simulink model "SystemPIDClosedLoop_motor_closed_zrate_js"  (Simulink 7.7)
settings: Solver=ode4  StartTime=0.0  StopTime=60  FixedStep=0.001  RelTol=1e-3
libraries: simulink x5, aerolibanimutils x1, aerolibfltsims x1
settings Model: Creator=Rakhi  LastModifiedBy=Rakhi
settings SolverCC: PositivePriorityOrder=on

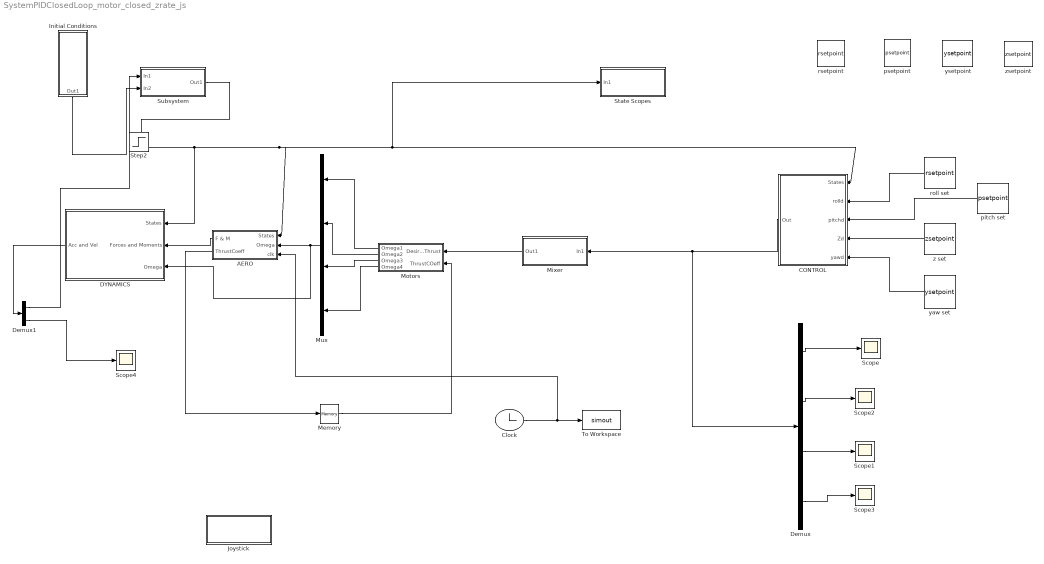
== system SystemPIDClosedLoop_motor_closed_zrate_js ==
  AERO : Subsystem
  CONTROL : Subsystem
      settings: AttributesFormatString=%<Priority>
  Clock : Clock
  DYNAMICS : Subsystem
  Demux : Demux
  Demux1 : Demux  Outputs=[12 1]
  Initial Conditions : Subsystem
  Joystick : Subsystem
  Memory : Memory  X0=3.1751e-5  InheritSampleTime=on
  Mixer : Subsystem
  Motors : Subsystem
  Mux : Mux
  Scope{,1..4} (5 alike) : Scope
      Scope settings: YMin=-900  YMax=-50
      Scope1 settings: YMin=-30  YMax=30
      Scope2 settings: SaveName=ScopeData2
      Scope3 settings: SaveName=ScopeData3
      Scope4 settings: SaveName=ScopeData4
  State Scopes : Subsystem
  Subsystem : Subsystem
  To Workspace : ToWorkspace  VariableName=simout  SampleTime=-1  SaveFormat=Structure
      settings: MaxDataPoints=1
  pitch set : DataStoreRead  DataStoreName=psetpoint  SampleTime=0.001  DataStoreElements=psetpoint
  psetpoint : DataStoreMemory  DataStoreName=psetpoint
  roll set : DataStoreRead  DataStoreName=rsetpoint  SampleTime=0.001  DataStoreElements=rsetpoint
  rsetpoint : DataStoreMemory  DataStoreName=rsetpoint
  yaw set : DataStoreRead  DataStoreName=ysetpoint  SampleTime=0.001  DataStoreElements=ysetpoint
  ysetpoint : DataStoreMemory  DataStoreName=ysetpoint
  z set : DataStoreRead  DataStoreName=zsetpoint  SampleTime=0.001  DataStoreElements=zsetpoint
  zsetpoint : DataStoreMemory  DataStoreName=zsetpoint  InitialValue=-45
  Step2 : Step  IOType=siggen  SampleTime=0
  wires:
  AERO/1(F & M) -> DYNAMICS/2(Forces and Moments)
  Initial Conditions/1(Out1) -> Subsystem/2(In2)
  Subsystem/1(Out1) -> DYNAMICS/1(States), AERO/1(States), CONTROL/1(States), State Scopes/1(In1)
  Demux/1 -> Scope/1
  Demux/2 -> Scope2/1
  Demux/4 -> Scope3/1
  CONTROL/1(Out) -> Mixer/1(In1), Demux/1
  Demux1/1 -> Subsystem/1(In1)
  DYNAMICS/1(Acc and Vel) -> Demux1/1
  Demux1/2 -> Scope4/1
  Clock/1 -> To Workspace/1, AERO/3(clk)
  Mux/1 -> AERO/2(Omega), DYNAMICS/3(Omega)
  Demux/3 -> Scope1/1
  AERO/2(ThrustCoeff) -> Memory/1
  Mixer/1(Out1) -> Motors/1(DesiredThrust)
  Memory/1 -> Motors/2(ThrustCOeff)
  Motors/1(Omega1) -> Mux/1
  Motors/2(Omega2) -> Mux/2
  Motors/3(Omega3) -> Mux/3
  Motors/4(Omega4) -> Mux/4
  roll set/1 -> CONTROL/2(rolld)
  pitch set/1 -> CONTROL/3(pitchd)
  z set/1 -> CONTROL/4(Zd)
  yaw set/1 -> CONTROL/5(yawd)

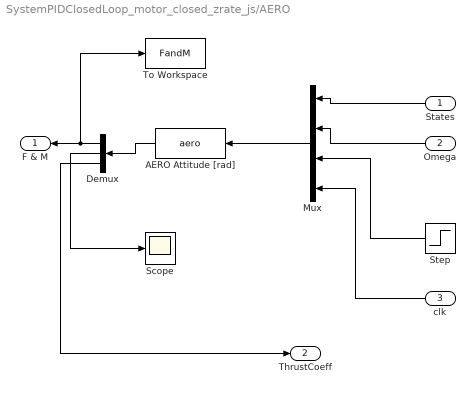
== system SystemPIDClosedLoop_motor_closed_zrate_js/AERO ==
  States : Inport
  Omega : Inport  Port=2
  clk : Inport  Port=3
  AERO Attitude [rad] : MATLABFcn  MATLABFcn=aero  OutputDimensions=26
  Demux : Demux  Outputs=[24 1 1]
  Mux : Mux
  Scope : Scope
      settings: SaveName=ScopeData5
  Step : Step  Time=0  Before=4  After=4  SampleTime=0
  To Workspace : ToWorkspace  VariableName=FandM  SampleTime=-1  SaveFormat=Structure
      settings: MaxDataPoints=1
  F & M : Outport
  ThrustCoeff : Outport  Port=2
  wires:
  Step/1 -> Mux/3
  Omega/1 -> Mux/2
  States/1 -> Mux/1
  Mux/1 -> AERO Attitude [rad]/1
  clk/1 -> Mux/4
  AERO Attitude [rad]/1 -> Demux/1
  Demux/1 -> F & M/1, To Workspace/1
  Demux/2 -> Scope/1
  Demux/3 -> ThrustCoeff/1

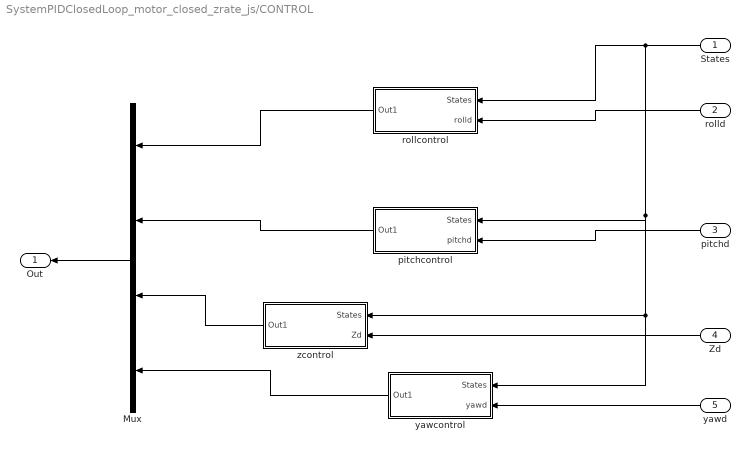
== system SystemPIDClosedLoop_motor_closed_zrate_js/CONTROL ==
  States : Inport
  rolld : Inport  Port=2
  pitchd : Inport  Port=3
  Zd : Inport  Port=4
  yawd : Inport  Port=5
  Mux : Mux
  pitchcontrol : Subsystem
  rollcontrol : Subsystem
  yawcontrol : Subsystem
  zcontrol : Subsystem
  Out : Outport
  wires:
  States/1 -> rollcontrol/1(States), pitchcontrol/1(States), yawcontrol/1(States), zcontrol/1(States)
  rolld/1 -> rollcontrol/2(rolld)
  pitchd/1 -> pitchcontrol/2(pitchd)
  yawd/1 -> yawcontrol/2(yawd)
  Zd/1 -> zcontrol/2(Zd)
  rollcontrol/1(Out1) -> Mux/1
  pitchcontrol/1(Out1) -> Mux/2
  zcontrol/1(Out1) -> Mux/3
  yawcontrol/1(Out1) -> Mux/4
  Mux/1 -> Out/1

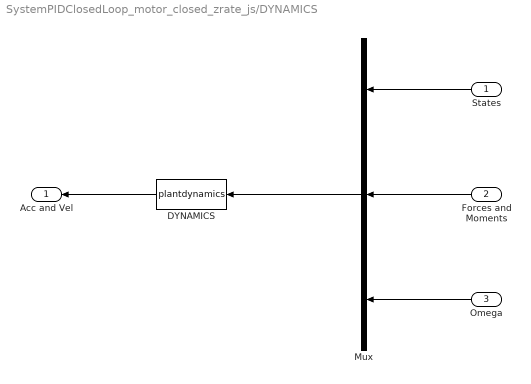
== system SystemPIDClosedLoop_motor_closed_zrate_js/DYNAMICS ==
  States : Inport
  Forces and Moments : Inport  Port=2
  Omega : Inport  Port=3
  DYNAMICS : MATLABFcn  MATLABFcn=plantdynamics  OutputDimensions=13
  Mux : Mux  Inputs=3
  Acc and Vel : Outport
  wires:
  States/1 -> Mux/1
  Forces and Moments/1 -> Mux/2
  Omega/1 -> Mux/3
  Mux/1 -> DYNAMICS/1
  DYNAMICS/1 -> Acc and Vel/1

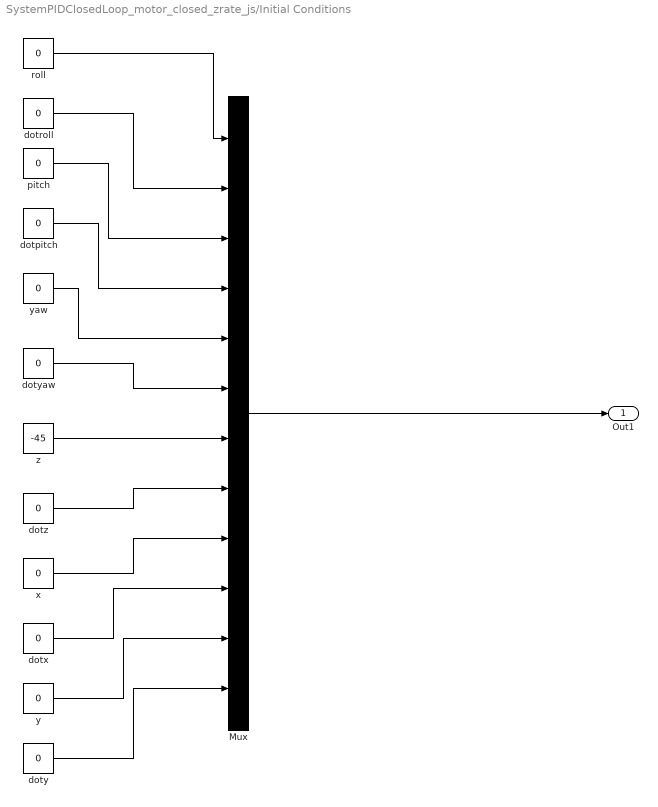
== system SystemPIDClosedLoop_motor_closed_zrate_js/Initial Conditions ==
  Mux : Mux  Inputs=12
  dotpitch : Constant  Value=0
  dotroll : Constant  Value=0
  dotx : Constant  Value=0
  doty : Constant  Value=0
  dotyaw : Constant  Value=0
  dotz : Constant  Value=0
  pitch : Constant  Value=0
  roll : Constant  Value=0
  x : Constant  Value=0
  y : Constant  Value=0
  yaw : Constant  Value=0
  z : Constant  Value=-45
  Out1 : Outport
  wires:
  doty/1 -> Mux/12
  y/1 -> Mux/11
  dotx/1 -> Mux/10
  x/1 -> Mux/9
  dotz/1 -> Mux/8
  z/1 -> Mux/7
  dotyaw/1 -> Mux/6
  yaw/1 -> Mux/5
  dotpitch/1 -> Mux/4
  pitch/1 -> Mux/3
  dotroll/1 -> Mux/2
  roll/1 -> Mux/1
  Mux/1 -> Out1/1

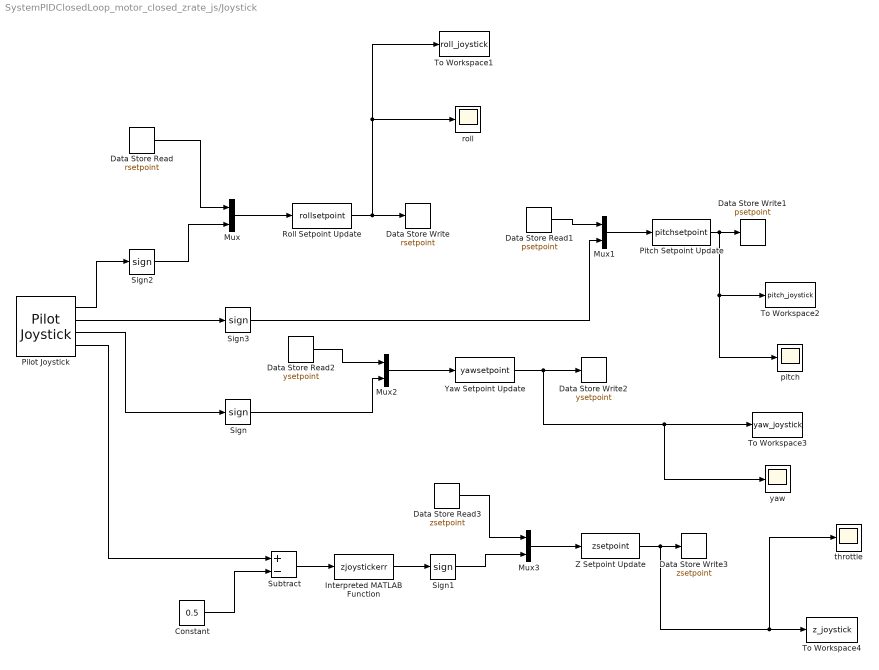
== system SystemPIDClosedLoop_motor_closed_zrate_js/Joystick ==
  Constant : Constant  Value=0.5
  Data Store Read : DataStoreRead  DataStoreName=rsetpoint  SampleTime=0.001  DataStoreElements=rsetpoint
  Data Store Read1 : DataStoreRead  DataStoreName=psetpoint  SampleTime=0.001  DataStoreElements=psetpoint
  Data Store Read2 : DataStoreRead  DataStoreName=ysetpoint  SampleTime=0.001  DataStoreElements=ysetpoint
  Data Store Read3 : DataStoreRead  DataStoreName=zsetpoint  SampleTime=.001  DataStoreElements=zsetpoint
  Data Store Write : DataStoreWrite  DataStoreName=rsetpoint  SampleTime=0.001  DataStoreElements=rsetpoint
  Data Store Write1 : DataStoreWrite  DataStoreName=psetpoint  SampleTime=0.001  DataStoreElements=psetpoint
  Data Store Write2 : DataStoreWrite  DataStoreName=ysetpoint  SampleTime=0.001  DataStoreElements=ysetpoint
  Data Store Write3 : DataStoreWrite  DataStoreName=zsetpoint  SampleTime=.001  DataStoreElements=zsetpoint
  Interpreted MATLAB Function : MATLABFcn  MATLABFcn=zjoystickerr
  Mux{,1..3} (4 alike) : Mux  Inputs=2
  Pilot Joystick : aerolibanimutils/Pilot Joystick  JoystickID=Joystick1  OutputConfiguration=FourAxis  SampleTime=0.001
  Pitch Setpoint Update : MATLABFcn  MATLABFcn=pitchsetpoint
  Roll Setpoint Update : MATLABFcn  MATLABFcn=rollsetpoint
  Sign{,1..3} (4 alike) : Signum
  Subtract : Sum  Inputs=+-
  To Workspace1 : ToWorkspace  VariableName=roll_joystick  SampleTime=-1  SaveFormat=Array
      settings: MaxDataPoints=1
  To Workspace2 : ToWorkspace  VariableName=pitch_joystick  SampleTime=-1  SaveFormat=Array
      settings: MaxDataPoints=1
  To Workspace3 : ToWorkspace  VariableName=yaw_joystick  SampleTime=-1  SaveFormat=Array
      settings: MaxDataPoints=1
  To Workspace4 : ToWorkspace  VariableName=z_joystick  SampleTime=-1  SaveFormat=Array
      settings: MaxDataPoints=1
  Yaw Setpoint Update : MATLABFcn  MATLABFcn=yawsetpoint
  Z Setpoint Update : MATLABFcn  MATLABFcn=zsetpoint
  pitch : Scope
      settings: YMin=-1  YMax=1  SaveName=ScopeData19
  roll : Scope
      settings: YMin=-1.5  YMax=1.5  SaveName=ScopeData21
  throttle : Scope
      settings: YMin=-49.5  YMax=-42.5  SaveName=ScopeData22
  yaw : Scope
      settings: YMin=-1.5  YMax=1.5  SaveName=ScopeData23
  wires:
  Pilot Joystick/3 -> Sign/1
  Constant/1 -> Subtract/2
  Pilot Joystick/4 -> Subtract/1
  Subtract/1 -> Interpreted MATLAB Function/1
  Interpreted MATLAB Function/1 -> Sign1/1
  Pilot Joystick/1 -> Sign2/1
  Pilot Joystick/2 -> Sign3/1
  Mux/1 -> Roll Setpoint Update/1
  Data Store Read/1 -> Mux/1
  Sign2/1 -> Mux/2
  Roll Setpoint Update/1 -> Data Store Write/1, To Workspace1/1, roll/1
  Data Store Read1/1 -> Mux1/1
  Sign3/1 -> Mux1/2
  Mux1/1 -> Pitch Setpoint Update/1
  Pitch Setpoint Update/1 -> Data Store Write1/1, To Workspace2/1, pitch/1
  Data Store Read2/1 -> Mux2/1
  Sign/1 -> Mux2/2
  Mux2/1 -> Yaw Setpoint Update/1
  Yaw Setpoint Update/1 -> Data Store Write2/1, To Workspace3/1, yaw/1
  Sign1/1 -> Mux3/2
  Data Store Read3/1 -> Mux3/1
  Mux3/1 -> Z Setpoint Update/1
  Z Setpoint Update/1 -> Data Store Write3/1, To Workspace4/1, throttle/1

== system SystemPIDClosedLoop_motor_closed_zrate_js/Mixer ==
  In1 : Inport
  Interpreted MATLAB Function : MATLABFcn  MATLABFcn=mix  OutputDimensions=4
  Out1 : Outport
  wires:
  In1/1 -> Interpreted MATLAB Function/1
  Interpreted MATLAB Function/1 -> Out1/1

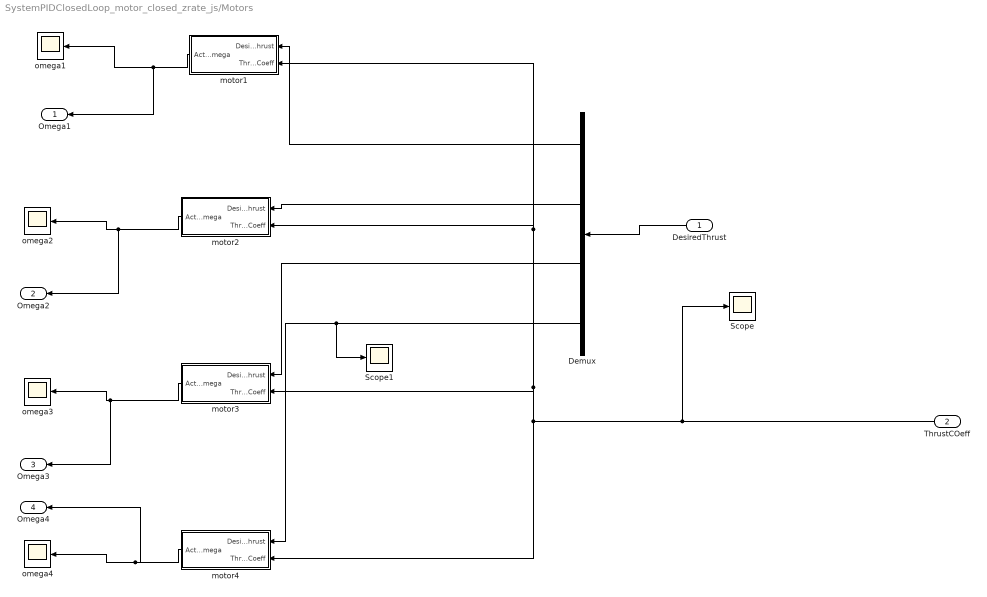
== system SystemPIDClosedLoop_motor_closed_zrate_js/Motors ==
  DesiredThrust : Inport
  ThrustCOeff : Inport  Port=2
  Demux : Demux
  Scope : Scope
      settings: SaveName=ScopeData7
  Scope1 : Scope
      settings: SaveName=ScopeData26
  motor1 : Subsystem
  motor2 : Subsystem
  motor3 : Subsystem
  motor4 : Subsystem
  omega{1..4} (4 alike) : Scope
      omega1 settings: YMin=-1  SaveName=ScopeData9
      omega2 settings: YMax=1  SaveName=ScopeData11
      omega3 settings: YMax=1  SaveName=ScopeData18
      omega4 settings: YMax=1  SaveName=ScopeData20
  Omega1 : Outport
  Omega2 : Outport  Port=2
  Omega3 : Outport  Port=3
  Omega4 : Outport  Port=4
  wires:
  DesiredThrust/1 -> Demux/1
  motor1/1(Actual Omega) -> Omega1/1, omega1/1
  motor2/1(Actual Omega) -> omega2/1, Omega2/1
  motor3/1(Actual Omega) -> omega3/1, Omega3/1
  motor4/1(Actual Omega) -> omega4/1, Omega4/1
  Demux/1 -> motor1/1(DesiredThrust)
  ThrustCOeff/1 -> motor1/2(ThrustCoeff), motor2/2(ThrustCoeff), motor3/2(ThrustCoeff), motor4/2(ThrustCoeff), Scope/1
  Demux/2 -> motor2/1(DesiredThrust)
  Demux/3 -> motor3/1(DesiredThrust)
  Demux/4 -> motor4/1(DesiredThrust), Scope1/1

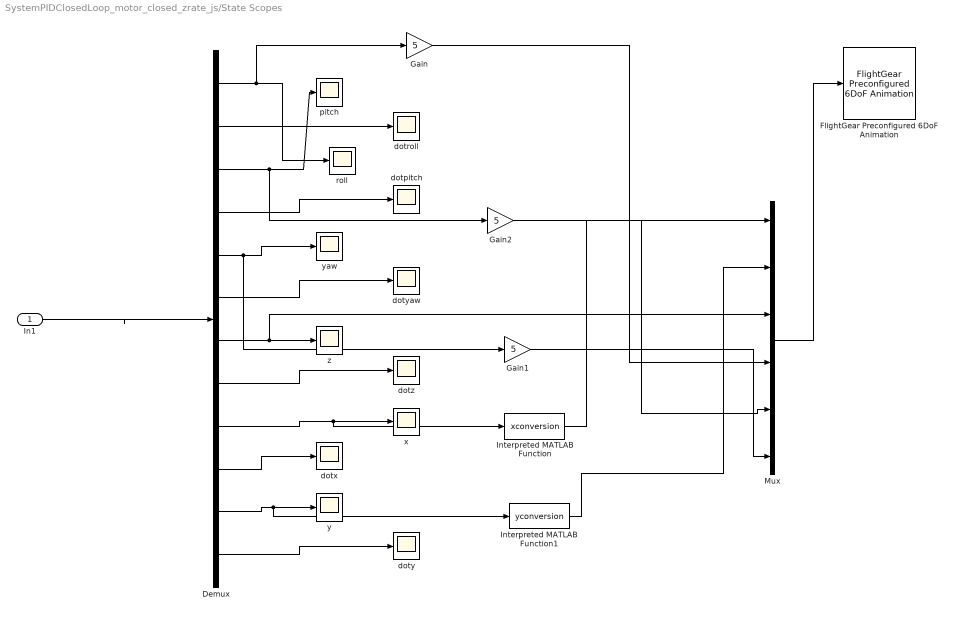
== system SystemPIDClosedLoop_motor_closed_zrate_js/State Scopes ==
  In1 : Inport
  Demux : Demux  Outputs=12
  FlightGear Preconfigured 6DoF Animation : aerolibfltsims/FlightGear Preconfigured 6DoF Animation  SystemSampleTime=-1  xFlightGearVersion=v0.9.8  DestinationIpAddress=127.0.0.1  DestinationPort=5502  SampleTime=-1
  Gain : Gain  Gain=5
  Gain1 : Gain  Gain=5
  Gain2 : Gain  Gain=5
  Interpreted MATLAB Function : MATLABFcn  MATLABFcn=xconversion
  Interpreted MATLAB Function1 : MATLABFcn  MATLABFcn=yconversion
  Mux : Mux  Inputs=6
  dotpitch : Scope
      settings: SaveName=ScopeData8
  dotroll : Scope
      settings: SaveName=ScopeData6
  dotx : Scope
      settings: SaveName=ScopeData14
  doty : Scope
      settings: SaveName=ScopeData16
  dotyaw : Scope
      settings: SaveName=ScopeData10
  dotz : Scope
      settings: SaveName=ScopeData12
  pitch : Scope
      settings: YMin=-0.5  YMax=0.5  SaveName=sc_pitch  DataFormat=Array
  roll : Scope
      settings: YMin=-0.0325  YMax=0  SaveName=sc_roll  DataFormat=Array
  x : Scope
      settings: SaveName=ScopeData13
  y : Scope
      settings: TimeRange=0.7999999999999972  YMin=-470.8125  YMax=-454.8125  SaveName=ScopeData15
  yaw : Scope
      settings: YMin=-0.5  YMax=0.1  SaveName=sc_yaw  DataFormat=Array
  z : Scope
      settings: YMin=-45  YMax=-44.2  SaveName=sc_z  DataFormat=Array
  wires:
  In1/1 -> Demux/1
  Demux/1 -> roll/1, Gain/1
  Demux/2 -> dotroll/1
  Demux/3 -> pitch/1, Gain2/1
  Demux/4 -> dotpitch/1
  Demux/5 -> yaw/1, Gain1/1
  Demux/6 -> dotyaw/1
  Demux/7 -> Mux/3, z/1
  Demux/8 -> dotz/1
  Demux/9 -> x/1, Interpreted MATLAB Function/1
  Demux/10 -> dotx/1
  Demux/11 -> y/1, Interpreted MATLAB Function1/1
  Demux/12 -> doty/1
  Interpreted MATLAB Function1/1 -> Mux/2
  Interpreted MATLAB Function/1 -> Mux/1
  Mux/1 -> FlightGear Preconfigured 6DoF Animation/1
  Gain/1 -> Mux/4
  Gain2/1 -> Mux/5
  Gain1/1 -> Mux/6

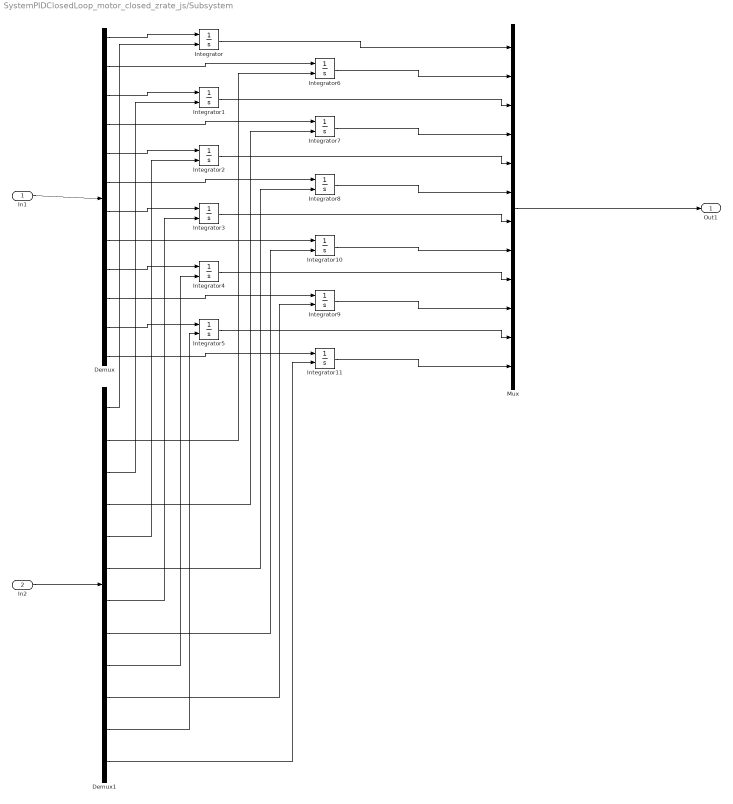
== system SystemPIDClosedLoop_motor_closed_zrate_js/Subsystem ==
  In1 : Inport
  In2 : Inport  Port=2
  Demux : Demux  Outputs=12
  Demux1 : Demux  Outputs=12
  Integrator{,1..11} (12 alike) : Integrator  InitialConditionSource=external
  Mux : Mux  Inputs=12
  Out1 : Outport
  wires:
  Demux/1 -> Integrator/1
  Demux/2 -> Integrator6/1
  Demux/3 -> Integrator1/1
  Demux/4 -> Integrator7/1
  Demux/5 -> Integrator2/1
  Demux/6 -> Integrator8/1
  Demux/7 -> Integrator3/1
  Demux/8 -> Integrator10/1
  Demux/9 -> Integrator4/1
  Demux/10 -> Integrator9/1
  Demux/11 -> Integrator5/1
  Demux/12 -> Integrator11/1
  In1/1 -> Demux/1
  Demux1/1 -> Integrator/2
  Demux1/2 -> Integrator6/2
  Demux1/3 -> Integrator1/2
  Demux1/4 -> Integrator7/2
  Demux1/5 -> Integrator2/2
  Demux1/6 -> Integrator8/2
  Demux1/7 -> Integrator3/2
  Demux1/8 -> Integrator10/2
  Demux1/9 -> Integrator4/2
  Demux1/10 -> Integrator9/2
  Demux1/11 -> Integrator5/2
  Demux1/12 -> Integrator11/2
  In2/1 -> Demux1/1
  Integrator/1 -> Mux/1
  Integrator6/1 -> Mux/2
  Integrator1/1 -> Mux/3
  Integrator7/1 -> Mux/4
  Integrator2/1 -> Mux/5
  Integrator8/1 -> Mux/6
  Integrator3/1 -> Mux/7
  Integrator10/1 -> Mux/8
  Integrator4/1 -> Mux/9
  Integrator9/1 -> Mux/10
  Integrator5/1 -> Mux/11
  Integrator11/1 -> Mux/12
  Mux/1 -> Out1/1

== system SystemPIDClosedLoop_motor_closed_zrate_js/CONTROL/pitchcontrol ==
  States : Inport
  pitchd : Inport  Port=2
  Interpreted MATLAB Function : MATLABFcn  MATLABFcn=pitcherr  OutputDimensions=1
  Mux : Mux  Inputs=2
  PID Controller : simulink/Continuous/PID Controller  SystemSampleTime=-1  Controller=PID  TimeDomain=Continuous-time  SampleTime=1  IntegratorMethod=Forward Euler  FilterMethod=Forward Euler  Form=Parallel  P=0.005  I=0  D=0.025  N=25  InitialConditionSource=internal  InitialConditionForIntegrator=0  InitialConditionForFilter=0  ExternalReset=none  LimitOutput=off  UpperSaturationLimit=inf  LowerSaturationLimit=-inf  LinearizeAsGain=off  AntiWindupMode=none  Kb=1  TrackingMode=off  Kt=1  PParamMin=[]  PParamMax=[]  IParamMin=[]  IParamMax=[]  DParamMin=[]  DParamMax=[]  NParamMin=[]  NParamMax=[]  KbParamMin=[]  KbParamMax=[]  KtParamMin=[]  KtParamMax=[]  POutMin=[]  POutMax=[]  IOutMin=[]  IOutMax=[]  DOutMin=[]  DOutMax=[]  NOutMin=[]  NOutMax=[]  KbOutMin=[]  KbOutMax=[]  KtOutMin=[]  KtOutMax=[]  IntegratorOutMin=[]  IntegratorOutMax=[]  FilterOutMin=[]  FilterOutMax=[]  SumOutMin=[]  SumOutMax=[]  SumI1OutMin=[]  SumI1OutMax=[]  SumI2OutMin=[]  SumI2OutMax=[]  SumI3OutMin=[]  SumI3OutMax=[]  SumDOutMin=[]  SumDOutMax=[]  SaturationOutMin=[]  SaturationOutMax=[]  IntegratorContinuousStateAttributes=''  IntegratorStateMustResolveToSignalObject=off  IntegratorRTWStateStorageClass=Auto  FilterContinuousStateAttributes=''  FilterStateMustResolveToSignalObject=off  FilterRTWStateStorageClass=Auto
  Out1 : Outport
  wires:
  States/1 -> Mux/1
  pitchd/1 -> Mux/2
  Mux/1 -> Interpreted MATLAB Function/1
  Interpreted MATLAB Function/1 -> PID Controller/1
  PID Controller/1 -> Out1/1

== system SystemPIDClosedLoop_motor_closed_zrate_js/CONTROL/rollcontrol ==
  States : Inport
  rolld : Inport  Port=2
  Interpreted MATLAB Function : MATLABFcn  MATLABFcn=rollerr  OutputDimensions=1
  Mux : Mux  Inputs=2
  PID Controller : simulink/Continuous/PID Controller  SystemSampleTime=-1  Controller=PID  TimeDomain=Continuous-time  SampleTime=1  IntegratorMethod=Forward Euler  FilterMethod=Forward Euler  Form=Parallel  P=.005  I=0  D=.025  N=25  InitialConditionSource=internal  InitialConditionForIntegrator=0  InitialConditionForFilter=0  ExternalReset=none  LimitOutput=off  UpperSaturationLimit=inf  LowerSaturationLimit=-inf  LinearizeAsGain=off  AntiWindupMode=none  Kb=1  TrackingMode=off  Kt=1  PParamMin=[]  PParamMax=[]  IParamMin=[]  IParamMax=[]  DParamMin=[]  DParamMax=[]  NParamMin=[]  NParamMax=[]  KbParamMin=[]  KbParamMax=[]  KtParamMin=[]  KtParamMax=[]  POutMin=[]  POutMax=[]  IOutMin=[]  IOutMax=[]  DOutMin=[]  DOutMax=[]  NOutMin=[]  NOutMax=[]  KbOutMin=[]  KbOutMax=[]  KtOutMin=[]  KtOutMax=[]  IntegratorOutMin=[]  IntegratorOutMax=[]  FilterOutMin=[]  FilterOutMax=[]  SumOutMin=[]  SumOutMax=[]  SumI1OutMin=[]  SumI1OutMax=[]  SumI2OutMin=[]  SumI2OutMax=[]  SumI3OutMin=[]  SumI3OutMax=[]  SumDOutMin=[]  SumDOutMax=[]  SaturationOutMin=[]  SaturationOutMax=[]  IntegratorContinuousStateAttributes=''  IntegratorStateMustResolveToSignalObject=off  IntegratorRTWStateStorageClass=Auto  FilterContinuousStateAttributes=''  FilterStateMustResolveToSignalObject=off  FilterRTWStateStorageClass=Auto
  Out1 : Outport
  wires:
  States/1 -> Mux/1
  rolld/1 -> Mux/2
  Mux/1 -> Interpreted MATLAB Function/1
  Interpreted MATLAB Function/1 -> PID Controller/1
  PID Controller/1 -> Out1/1

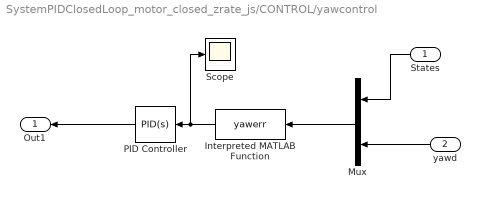
== system SystemPIDClosedLoop_motor_closed_zrate_js/CONTROL/yawcontrol ==
  States : Inport
  yawd : Inport  Port=2
  Interpreted MATLAB Function : MATLABFcn  MATLABFcn=yawerr  OutputDimensions=1
  Mux : Mux  Inputs=2
  PID Controller : simulink/Continuous/PID Controller  SystemSampleTime=-1  Controller=PID  TimeDomain=Continuous-time  SampleTime=1  IntegratorMethod=Forward Euler  FilterMethod=Forward Euler  Form=Parallel  P=0.05  I=0  D=0.25  N=25  InitialConditionSource=internal  InitialConditionForIntegrator=0  InitialConditionForFilter=0  ExternalReset=none  LimitOutput=off  UpperSaturationLimit=inf  LowerSaturationLimit=-inf  LinearizeAsGain=off  AntiWindupMode=none  Kb=1  TrackingMode=off  Kt=1  PParamMin=[]  PParamMax=[]  IParamMin=[]  IParamMax=[]  DParamMin=[]  DParamMax=[]  NParamMin=[]  NParamMax=[]  KbParamMin=[]  KbParamMax=[]  KtParamMin=[]  KtParamMax=[]  POutMin=[]  POutMax=[]  IOutMin=[]  IOutMax=[]  DOutMin=[]  DOutMax=[]  NOutMin=[]  NOutMax=[]  KbOutMin=[]  KbOutMax=[]  KtOutMin=[]  KtOutMax=[]  IntegratorOutMin=[]  IntegratorOutMax=[]  FilterOutMin=[]  FilterOutMax=[]  SumOutMin=[]  SumOutMax=[]  SumI1OutMin=[]  SumI1OutMax=[]  SumI2OutMin=[]  SumI2OutMax=[]  SumI3OutMin=[]  SumI3OutMax=[]  SumDOutMin=[]  SumDOutMax=[]  SaturationOutMin=[]  SaturationOutMax=[]  IntegratorContinuousStateAttributes=''  IntegratorStateMustResolveToSignalObject=off  IntegratorRTWStateStorageClass=Auto  FilterContinuousStateAttributes=''  FilterStateMustResolveToSignalObject=off  FilterRTWStateStorageClass=Auto
  Scope : Scope
      settings: SaveName=ScopeData17
  Out1 : Outport
  wires:
  States/1 -> Mux/1
  yawd/1 -> Mux/2
  Mux/1 -> Interpreted MATLAB Function/1
  Interpreted MATLAB Function/1 -> PID Controller/1, Scope/1
  PID Controller/1 -> Out1/1

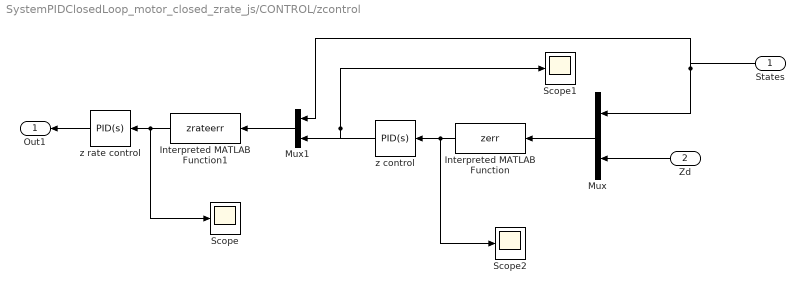
== system SystemPIDClosedLoop_motor_closed_zrate_js/CONTROL/zcontrol ==
  States : Inport
  Zd : Inport  Port=2
  Interpreted MATLAB Function : MATLABFcn  MATLABFcn=zerr  OutputDimensions=1
  Interpreted MATLAB Function1 : MATLABFcn  MATLABFcn=zrateerr
  Mux : Mux  Inputs=2
  Mux1 : Mux  Inputs=2
  Scope : Scope
      settings: SaveName=ScopeData25
  Scope1 : Scope
      settings: YMin=-30  YMax=30  SaveName=ScopeData24
  Scope2 : Scope
      settings: SaveName=ScopeData27
  z control : simulink/Continuous/PID Controller  SystemSampleTime=-1  Controller=PID  TimeDomain=Continuous-time  SampleTime=1  IntegratorMethod=Forward Euler  FilterMethod=Forward Euler  Form=Parallel  P=1  I=0  D=0  N=100  InitialConditionSource=internal  InitialConditionForIntegrator=0  InitialConditionForFilter=0  ExternalReset=none  LimitOutput=on  UpperSaturationLimit=2.5  LowerSaturationLimit=-2.5  LinearizeAsGain=off  AntiWindupMode=clamping  Kb=1  TrackingMode=off  Kt=1  PParamMin=[]  PParamMax=[]  IParamMin=[]  IParamMax=[]  DParamMin=[]  DParamMax=[]  NParamMin=[]  NParamMax=[]  KbParamMin=[]  KbParamMax=[]  KtParamMin=[]  KtParamMax=[]  POutMin=[]  POutMax=[]  IOutMin=[]  IOutMax=[]  DOutMin=[]  DOutMax=[]  NOutMin=[]  NOutMax=[]  KbOutMin=[]  KbOutMax=[]  KtOutMin=[]  KtOutMax=[]  IntegratorOutMin=[]  IntegratorOutMax=[]  FilterOutMin=[]  FilterOutMax=[]  SumOutMin=[]  SumOutMax=[]  SumI1OutMin=[]  SumI1OutMax=[]  SumI2OutMin=[]  SumI2OutMax=[]  SumI3OutMin=[]  SumI3OutMax=[]  SumDOutMin=[]  SumDOutMax=[]  SaturationOutMin=[]  SaturationOutMax=[]  IntegratorContinuousStateAttributes=''  IntegratorStateMustResolveToSignalObject=off  IntegratorRTWStateStorageClass=Auto  FilterContinuousStateAttributes=''  FilterStateMustResolveToSignalObject=off  FilterRTWStateStorageClass=Auto
  z rate control : simulink/Continuous/PID Controller  SystemSampleTime=-1  Controller=PID  TimeDomain=Continuous-time  SampleTime=1  IntegratorMethod=Forward Euler  FilterMethod=Forward Euler  Form=Parallel  P=5  I=2  D=4  N=100  InitialConditionSource=internal  InitialConditionForIntegrator=0  InitialConditionForFilter=0  ExternalReset=none  LimitOutput=off  UpperSaturationLimit=5  LowerSaturationLimit=-5  LinearizeAsGain=off  AntiWindupMode=clamping  Kb=1  TrackingMode=off  Kt=1  PParamMin=[]  PParamMax=[]  IParamMin=[]  IParamMax=[]  DParamMin=[]  DParamMax=[]  NParamMin=[]  NParamMax=[]  KbParamMin=[]  KbParamMax=[]  KtParamMin=[]  KtParamMax=[]  POutMin=[]  POutMax=[]  IOutMin=[]  IOutMax=[]  DOutMin=[]  DOutMax=[]  NOutMin=[]  NOutMax=[]  KbOutMin=[]  KbOutMax=[]  KtOutMin=[]  KtOutMax=[]  IntegratorOutMin=[]  IntegratorOutMax=[]  FilterOutMin=[]  FilterOutMax=[]  SumOutMin=[]  SumOutMax=[]  SumI1OutMin=[]  SumI1OutMax=[]  SumI2OutMin=[]  SumI2OutMax=[]  SumI3OutMin=[]  SumI3OutMax=[]  SumDOutMin=[]  SumDOutMax=[]  SaturationOutMin=[]  SaturationOutMax=[]  IntegratorContinuousStateAttributes=''  IntegratorStateMustResolveToSignalObject=off  IntegratorRTWStateStorageClass=Auto  FilterContinuousStateAttributes=''  FilterStateMustResolveToSignalObject=off  FilterRTWStateStorageClass=Auto
  Out1 : Outport
  wires:
  States/1 -> Mux/1, Mux1/1
  Zd/1 -> Mux/2
  Mux/1 -> Interpreted MATLAB Function/1
  Interpreted MATLAB Function/1 -> z control/1, Scope2/1
  z control/1 -> Scope1/1, Mux1/2
  Mux1/1 -> Interpreted MATLAB Function1/1
  Interpreted MATLAB Function1/1 -> Scope/1, z rate control/1
  z rate control/1 -> Out1/1

== system SystemPIDClosedLoop_motor_closed_zrate_js/Motors/motor1 ==
  DesiredThrust : Inport
  ThrustCoeff : Inport  Port=2
  Interpreted MATLAB Function : MATLABFcn  MATLABFcn=motor1
  Mux : Mux  Inputs=2
  Transfer Fcn : TransferFcn  Numerator=[0 0.936]  Denominator=[0.178 1]
  Actual Omega : Outport
  wires:
  DesiredThrust/1 -> Mux/1
  ThrustCoeff/1 -> Mux/2
  Mux/1 -> Interpreted MATLAB Function/1
  Interpreted MATLAB Function/1 -> Transfer Fcn/1
  Transfer Fcn/1 -> Actual Omega/1

== system SystemPIDClosedLoop_motor_closed_zrate_js/Motors/motor2 ==
  DesiredThrust : Inport
  ThrustCoeff : Inport  Port=2
  Interpreted MATLAB Function : MATLABFcn  MATLABFcn=motor2
  Mux : Mux  Inputs=2
  Transfer Fcn : TransferFcn  Numerator=[0 0.936]  Denominator=[0.178 1]
  Actual Omega : Outport
  wires:
  ThrustCoeff/1 -> Mux/2
  DesiredThrust/1 -> Mux/1
  Mux/1 -> Interpreted MATLAB Function/1
  Interpreted MATLAB Function/1 -> Transfer Fcn/1
  Transfer Fcn/1 -> Actual Omega/1

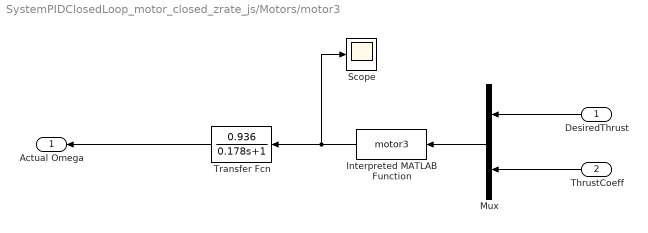
== system SystemPIDClosedLoop_motor_closed_zrate_js/Motors/motor3 ==
  DesiredThrust : Inport
  ThrustCoeff : Inport  Port=2
  Interpreted MATLAB Function : MATLABFcn  MATLABFcn=motor3
  Mux : Mux  Inputs=2
  Scope : Scope
      settings: SaveName=ScopeData28
  Transfer Fcn : TransferFcn  Numerator=[0 0.936]  Denominator=[0.178 1]
  Actual Omega : Outport
  wires:
  DesiredThrust/1 -> Mux/1
  ThrustCoeff/1 -> Mux/2
  Mux/1 -> Interpreted MATLAB Function/1
  Interpreted MATLAB Function/1 -> Transfer Fcn/1, Scope/1
  Transfer Fcn/1 -> Actual Omega/1

== system SystemPIDClosedLoop_motor_closed_zrate_js/Motors/motor4 ==
  DesiredThrust : Inport
  ThrustCoeff : Inport  Port=2
  Interpreted MATLAB Function : MATLABFcn  MATLABFcn=motor4
  Mux : Mux  Inputs=2
  Transfer Fcn : TransferFcn  Numerator=[0 0.936]  Denominator=[0.178 1]
  Actual Omega : Outport
  wires:
  DesiredThrust/1 -> Mux/1
  ThrustCoeff/1 -> Mux/2
  Mux/1 -> Interpreted MATLAB Function/1
  Interpreted MATLAB Function/1 -> Transfer Fcn/1
  Transfer Fcn/1 -> Actual Omega/1
